simulink model "Pendulum_Robot_Subsystem"  (R2015a)
settings: Solver=ode45  StartTime=0.0  StopTime=10.0  RelTol=1e-3
values from neighbouring files (symbols this model uses):
  b_phi = 0    [Setup_Parameters.m]
  b_x = 0    [Setup_Parameters.m]
  l = .38    (= 0.38)    [Setup_Parameters.m]
  m1 = .6    (= 0.6)    [Setup_Parameters.m]
  m2 = 1.9    [Setup_Parameters.m]
  r = Wheel_radius/39.37    (= 0.0762001524003)    [Setup_Parameters.m]
settings Model: Creator=tvincent  LastModifiedBy=tvincent

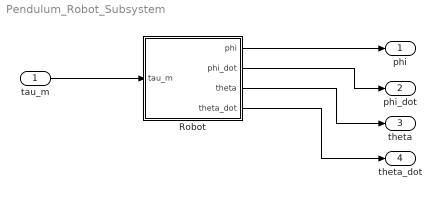
== system Pendulum_Robot_Subsystem ==
  tau_m : Inport
  Robot : Subsystem
  phi : Outport
  phi_dot : Outport  Port=2
  theta : Outport  Port=3
  theta_dot : Outport  Port=4
  wires:
  Robot/2(phi_dot) -> phi_dot/1
  Robot/3(theta) -> theta/1
  Robot/1(phi) -> phi/1
  Robot/4(theta_dot) -> theta_dot/1
  tau_m/1 -> Robot/1(tau_m)

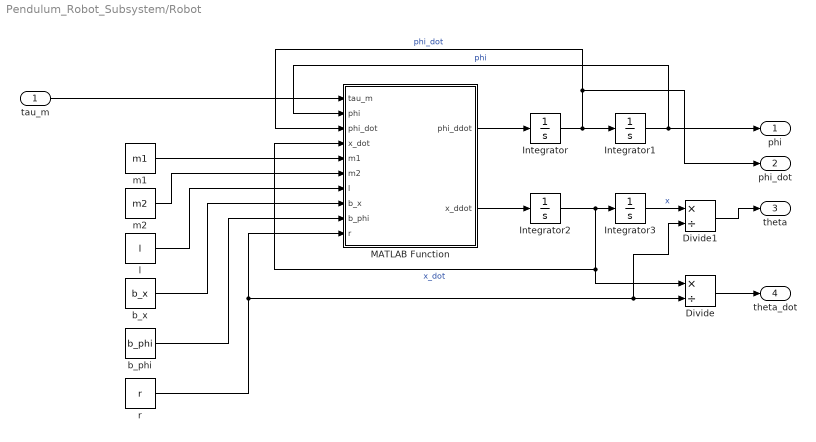
== system Pendulum_Robot_Subsystem/Robot ==
  tau_m : Inport
  Divide : Product  Inputs=*/
  Divide1 : Product  Inputs=*/
  Integrator{,1..3} (4 alike) : Integrator
  MATLAB Function : MATLAB Function  TreatAsAtomicUnit=on
  b_phi : Constant  Value=b_phi
  b_x : Constant  Value=b_x
  l : Constant  Value=l
  m1 : Constant  Value=m1
  m2 : Constant  Value=m2
  r : Constant  Value=r
  phi : Outport
  phi_dot : Outport  Port=2
  theta : Outport  Port=3
  theta_dot : Outport  Port=4
  wires:
  Integrator2/1 -> MATLAB Function/4(x_dot), Divide/1, Integrator3/1  "x_dot"
  m1/1 -> MATLAB Function/5(m1)
  Integrator1/1 -> phi/1, MATLAB Function/2(phi)  "phi"
  MATLAB Function/1(phi_ddot) -> Integrator/1
  MATLAB Function/2(x_ddot) -> Integrator2/1
  l/1 -> MATLAB Function/7(l)
  b_x/1 -> MATLAB Function/8(b_x)
  m2/1 -> MATLAB Function/6(m2)
  b_phi/1 -> MATLAB Function/9(b_phi)
  tau_m/1 -> MATLAB Function/1(tau_m)
  r/1 -> Divide1/2, Divide/2, MATLAB Function/10(r)
  Integrator/1 -> phi_dot/1, MATLAB Function/3(phi_dot), Integrator1/1  "phi_dot"
  Divide/1 -> theta_dot/1
  Integrator3/1 -> Divide1/1  "x"
  Divide1/1 -> theta/1

== matlab function Pendulum_Robot_Subsystem/Robot/MATLAB Function ==
  data: tau_m input; phi_ddot output; phi input; phi_dot input; x_dot input; m1 input; m2 input; l input; b_x input; b_phi input; r input; x_ddot output
function [phi_ddot,x_ddot] = phi_ddot(tau_m,phi,phi_dot,x_dot,m1,m2,l,b_x,b_phi,r)
%#codegen

g=9.81;

phi_ddot = ((g*(m1+m2) - m1*l*cos(phi)*(phi_dot)^2)*sin(phi) - cos(phi)*b_x*x_dot - ...
    ((m1+m2)/(m1*l))*b_phi*phi_dot + ((m1+m2)/(m1*l) + cos(phi)/r)*tau_m) / ...
    l*(m2+m1*sin(phi)^2);

x_ddot = (g*m1*cos(phi)*sin(phi) - m1*l*sin(phi)*phi_dot^2 - b_x*x_dot - ...
    cos(phi)*b_phi*phi_dot + (cos(phi)+(1/r))*tau_m) / ...
    (m2+m1*sin(phi)^2);
